simulink model "MCC"  (Simulink 9.0)
settings: Solver=ode15s  StartTime=0.0  StopTime=0.2  RelTol=1e-3
InitFcn:
  | MCC_constants
StartFcn:
  | MCC_constants
values from neighbouring files (symbols this model uses):
  b = 3.5077E-6    (= 3.5077e-06)    [MCC_constants.m]    (also in TD2_config.m = 0.0085)
  Cr = 0    [MCC_constants.m]
  J = 3.2248E-6    (= 3.2248e-06)    [MCC_constants.m]    (also in TD2_config.m = 0.28)
  K = 0.0274    [MCC_constants.m]    (also in TD2_config.m = 0.5093)
  L = 2.75E-6    (= 2.75e-06)    [MCC_constants.m]    (also in TD2_config.m = 0.0016)
  R = 4    [MCC_constants.m]    (also in TD2_config.m = 0.13)
settings Model: Creator=GEII Robot  LastModifiedBy=GEII Robot
settings DataIOCC: SaveFormat=Dataset
settings OptimizationCC: LifeSpan=auto
settings DebuggingCC: UnderspecifiedInitializationDetection=Simplified  MergeDetectMultiDrivingBlocksExec=error  SFUnexpectedBacktrackingDiag=error  SFNoUnconditionalDefaultTransitionDiag=error  SFExecutionAtInitializationDiag=warning
settings HardwareCC: ProdBitPerPointer=64  ProdBitPerSizeT=64  ProdBitPerPtrDiffT=64  ProdLargestAtomicFloat=Float  ProdIntDivRoundTo=Zero  ProdEndianess=LittleEndian  ProdWordSize=64  ProdHWDeviceType=Intel->x86-64 (Windows64)
settings ModelReferenceCC: PropagateSignalLabelsOutOfModel=on
settings CodeAppCC: StateflowObjectComments=off
settings GRTTargetCC: TargetLangStandard=C99 (ISO)
settings ConfigComp: CovMetricSettings=dwe  CovHtmlReporting=off  CovSaveCumulativeToWorkspaceVar=off  CovSaveSingleToWorkspaceVar=off  CovExternalEMLEnable=on

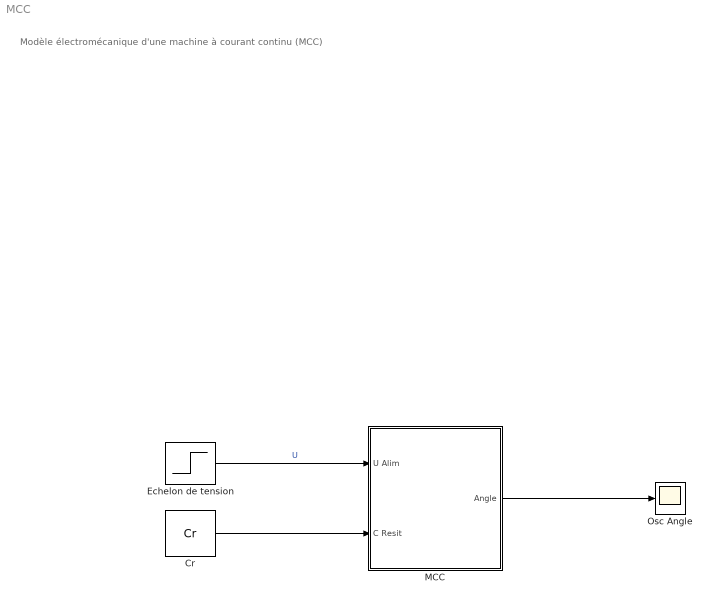
== system MCC ==
  note: Modèle électromécanique d'une machine à courant continu (MCC)
  Cr : Constant  Value=Cr
  Echelon de tension : Step  Time=0  After=12  SampleTime=0
  MCC : Subsystem
  Osc Angle : Scope
  wires:
  Echelon de tension/1 -> MCC/1(U Alim)  "U"
  Cr/1 -> MCC/2(C Resit)
  MCC/1(Angle) -> Osc Angle/1

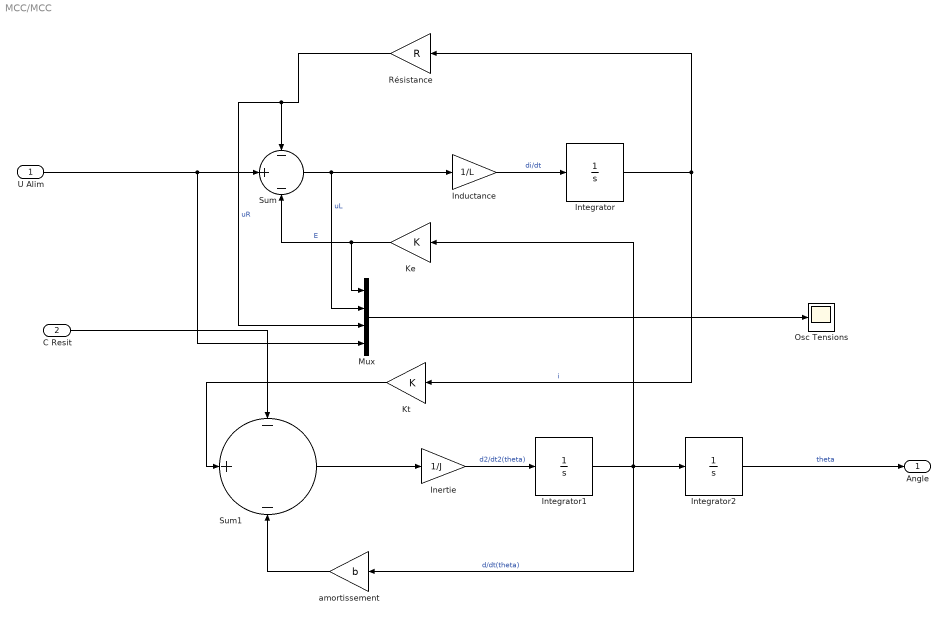
== system MCC/MCC ==
  U Alim : Inport
  C Resit : Inport  Port=2
  Inductance : Gain  Gain=1/L
  Inertie : Gain  Gain=1/J
  Integrator : Integrator
  Integrator1 : Integrator
  Integrator2 : Integrator
  Ke : Gain  Gain=K
  Kt : Gain  Gain=K
  Mux : Mux
  Osc Tensions : Scope
  Résistance : Gain  Gain=R
  Sum : Sum  Inputs=-|+|-
  Sum1 : Sum  Inputs=-|+|-
  amortissement : Gain  Gain=b
  Angle : Outport
  wires:
  Mux/1 -> Osc Tensions/1
  Sum1/1 -> Inertie/1
  Inertie/1 -> Integrator1/1  "d2/dt2(theta)"
  Integrator2/1 -> Angle/1  "theta"
  C Resit/1 -> Sum1/1
  amortissement/1 -> Sum1/3
  Ke/1 -> Mux/1, Sum/3  "E"
  U Alim/1 -> Mux/4, Sum/2
  Kt/1 -> Sum1/2
  Résistance/1 -> Mux/3, Sum/1  "uR"
  Integrator/1 -> Résistance/1, Kt/1  "i"
  Integrator1/1 -> amortissement/1, Ke/1, Integrator2/1  "d/dt(theta)"
  Sum/1 -> Inductance/1, Mux/2  "uL"
  Inductance/1 -> Integrator/1  "di/dt"
